simulink model "mbk"  (R2020a)
settings: Solver=ode4  StartTime=0.0  StopTime=10  FixedStep=0.01  RelTol=1e-3
InitFcn:
  | MBK
values from neighbouring files (symbols this model uses):
  b = 100    [Finder.m]    (also in MBK.m = 2; TCACS.m = Domain(2,:))
  k = 5    [MBK.m]
  m = 10    [MBK.m]
undefined symbols (not defined in the file or in its folder): G
settings Model: Creator=Ali  LastModifiedBy=Ali
settings DataIOCC: ReturnWorkspaceOutputs=off
settings DebuggingCC: ArithmeticOperatorsInVariantConditions=warning
settings SFSimCC: SimUseLocalCustomCode=off  CustomCodeUndefinedFunction=UseInterfaceOnly
settings RTWCC: RTWUseLocalCustomCode=off

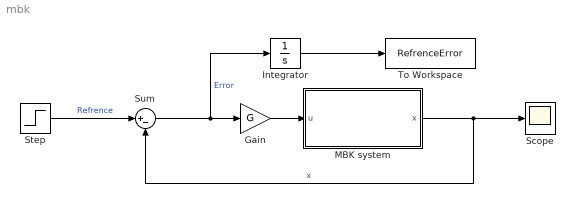
== system mbk ==
  Gain : Gain  Gain=G
  Integrator : Integrator
  MBK system : Subsystem
      mask Display: image('E:\Control\bachelor-thesis\Code\Simulink\MBK\MBKPic.png'); % Use "Edit Image" on toolstrip to change.
  Scope : Scope
  Step : Step  SampleTime=0
  Sum : Sum  Inputs=|+-
  To Workspace : ToWorkspace  VariableName=RefrenceError  SampleTime=-1
      settings: Save2DSignal=2-D array (concatenate along first dimension)
  wires:
  MBK system/1(x) -> Scope/1, Sum/2  "x"
  Gain/1 -> MBK system/1(u)
  Step/1 -> Sum/1  "Refrence"
  Sum/1 -> Integrator/1, Gain/1  "Error"
  Integrator/1 -> To Workspace/1

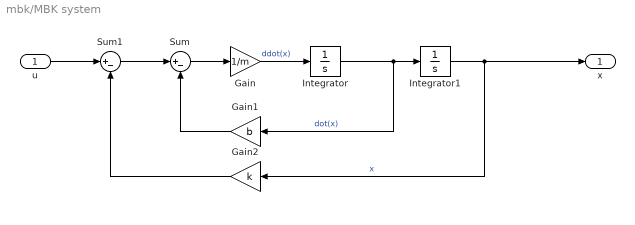
== system mbk/MBK system ==
  u : Inport
  Gain : Gain  Gain=1/m
  Gain1 : Gain  Gain=b
  Gain2 : Gain  Gain=k
  Integrator : Integrator
  Integrator1 : Integrator
  Sum : Sum  Inputs=|+-
  Sum1 : Sum  Inputs=|+-
  x : Outport
  wires:
  Integrator/1 -> Gain1/1, Integrator1/1  "dot(x)"
  Sum/1 -> Gain/1
  Sum1/1 -> Sum/1
  Gain2/1 -> Sum1/2
  Gain1/1 -> Sum/2
  Integrator1/1 -> x/1, Gain2/1  "x"
  Gain/1 -> Integrator/1  "ddot(x)"
  u/1 -> Sum1/1
